simulink library "Lib_Solve_DataOut_TMATS"  (R2015a)
settings: Solver=ode45  StartTime=0.0  StopTime=10.0  RelTol=1e-3
undefined symbols (not defined in the file): stripchar_TMATS
Description:
  | Thomas Modules
settings Model: CovSFcnEnable=off  Creator=jwchapm2  LastModifiedBy=jwchapm2
settings OptimizationCC: ExpressionDepthLimit=2147483647
settings DebuggingCC: UnderspecifiedInitializationDetection=Classic  MergeDetectMultiDrivingBlocksExec=none  SolverPrmCheckMsg=warning  StateNameClashWarn=warning

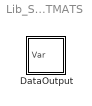
== system Lib_Solve_DataOut_TMATS ==
  DataOutput : Subsystem  mask(T-MATS: Data Output Library Block){FVar_M=double(strcat(stripchar_TMATS(gcb),'.bin'))}
      mask prompts: FVar_M "FVar_M - File name for Variable Output"
      mask help: This Block saves the input variable to a file at each time step. Note, this will overwrite the previous value.
      mask init:
      | FVar_M = double(FVar_M);
      mask Help: web(which('Solver_TMATS_DOut.html'),'-helpbrowser')

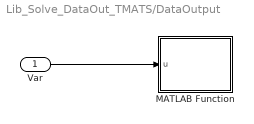
== system Lib_Solve_DataOut_TMATS/DataOutput ==
  Var : Inport
  MATLAB Function : MATLAB Function  TreatAsAtomicUnit=on
  wires:
  Var/1 -> MATLAB Function/1(u)

== matlab function Lib_Solve_DataOut_TMATS/DataOutput/MATLAB Function ==
  data: u input; FVar_M parameter
function fcn(u,FVar_M)
%#codegen
FileName = char(FVar_M);
FID = fopen(FileName,'w');
L = length(u);
for i = 1:L 
    u(i) = min(99999,u(i));
    fprintf(FID,'%f\n',u(i));
end
fclose(FID);
